simulink model "Tuning"  (R2022b)
settings: Solver=VariableStepAuto  StartTime=0.0  StopTime=100.03  RelTol=1e-3
undefined symbols (not defined in the file): A_matrix, B_matrix, C_matrix, D_matrix, dis_vec, rho_new, sigbuilder_block
libraries: slpidlib x1
settings Model: Creator=brianlesko  LastModifiedBy=brianlesko

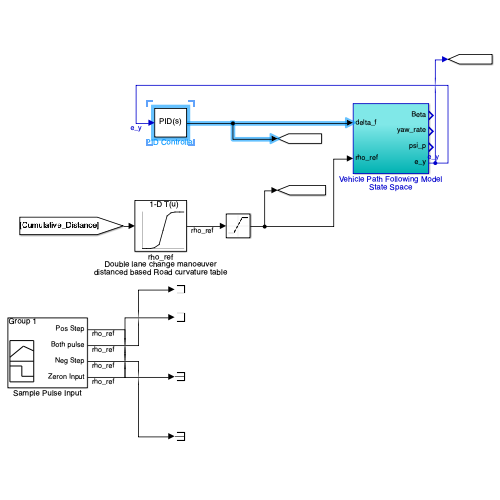
[thumbnail: Simulink's stored preview of the top-level diagram]
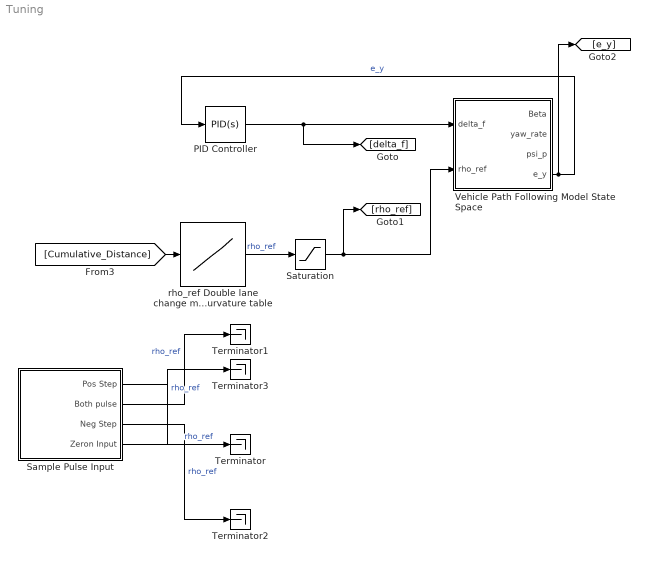
== system Tuning ==
  PID Controller : slpidlib/PID Controller  Controller=PID  Form=Parallel  TimeDomain=Continuous-time  UseExternalTs=off  SampleTime=-1  IntegratorMethod=Forward Euler  FilterMethod=Forward Euler  ControllerParametersSource=internal  P=1.6757e-08  I=1.1959e-08  UseKiTs=off  D=8.9738e-10  N=30  UseFilter=on  TunerSelectOption=Frequency Response Based  InitialConditionSource=internal  InitialConditionForIntegrator=0  InitialConditionForFilter=0  DifferentiatorICPrevScaledInput=0  ExternalReset=none  TrackingMode=off  Kt=1  LimitOutput=off  SatLimitsSource=internal  UpperSaturationLimit=inf  LowerSaturationLimit=-inf  LinearizeAsGain=on  AntiWindupMode=none  Kb=1  LimitIntegrator=off  UpperIntegratorSaturationLimit=inf  LowerIntegratorSaturationLimit=-inf  POutMin=[]  POutMax=[]  IOutMin=[]  IOutMax=[]  DOutMin=[]  DOutMax=[]  NOutMin=[]  NOutMax=[]  SumOutMin=[]  SumOutMax=[]  SaturationOutMin=[]  SaturationOutMax=[]  PParamMin=[]  PParamMax=[]  IParamMin=[]  IParamMax=[]  DParamMin=[]  DParamMax=[]  NParamMin=[]  NParamMax=[]  KbParamMin=[]  KbParamMax=[]  KtParamMin=[]  KtParamMax=[]  KbOutMin=[]  KbOutMax=[]  KtOutMin=[]  KtOutMax=[]  IntegratorOutMin=[]  IntegratorOutMax=[]  FilterOutMin=[]  FilterOutMax=[]  SumI1OutMin=[]  SumI1OutMax=[]  SumI2OutMin=[]  SumI2OutMax=[]  SumI3OutMin=[]  SumI3OutMax=[]  SumI4OutMin=[]  SumI4OutMax=[]  SumDOutMin=[]  SumDOutMax=[]  DifferentiatorOutMin=[]  DifferentiatorOutMax=[]  FilterDiffOutCoefMin=[]  FilterDiffOutCoefMax=[]  ReciprocalOutMin=[]  ReciprocalOutMax=[]  SumDenOutMin=[]  SumDenOutMax=[]  SumNumOutMin=[]  SumNumOutMax=[]  DivideOutMin=[]  DivideOutMax=[]  UdiffTsProdOutMin=[]  UdiffTsProdOutMax=[]  NTsProdOutMin=[]  NTsProdOutMax=[]  UintegralTsProdOutMin=[]  UintegralTsProdOutMax=[]  UngainTsProdOutMin=[]  UngainTsProdOutMax=[]  ClampingZeroOutDataTypeStr=Inherit: Inherit via back propagation  ClampingZeroOutMin=[]  ClampingZeroOutMax=[]  FilterDenConstantOutDataTypeStr=Inherit: Inherit via back propagation  FilterDenConstantOutMin=[]  FilterDenConstantOutMax=[]  PCopyOutDataTypeStr=Inherit: Inherit via back propagation  PCopyOutMin=[]  PCopyOutMax=[]  NCopyOutDataTypeStr=Inherit: Inherit via back propagation  NCopyOutMin=[]  NCopyOutMax=[]  IntegratorContinuousStateAttributes=''  IntegratorStateMustResolveToSignalObject=off  IntegratorRTWStateStorageClass=Auto  FilterContinuousStateAttributes=''  FilterStateMustResolveToSignalObject=off  FilterRTWStateStorageClass=Auto  ParallelPVariant=InternalParameters  IdealPVariant=Disabled  IVariant=InternalParameters  DVariant=InternalParameters  IntegratorVariant=Continuous  SatVariant=Disabled  AWVariant=Passthrough  PCopyVariant=Disabled  TRVariant=Disabled  FdbkBlocksVariant=Forward  IdealPFdbkVariant=Disabled  SatFdbkVariant=Disabled  DerivativeFilterVariant=ContFilter  NVariant=InternalParameters  NCopyVariant=Disabled  FilterICVariant=InternalICsFilter  IntegratorICVariant=InternalICs  ExternalResetVariant=Disabled  TRSumVariant=Passthrough  SumFdbkVariant=Disabled  SumVariant=Sum_PID  TsampFilterVariant=InternalTs  TsampNgainVariant=Passthrough  TsampIntegralVariant=Passthrough  ExternalSaturationOutDataTypeStr=Inherit: Same as second input
  Sample Pulse Input : Subsystem  Tag=STV Subsys  LoadFcn=sigbuilder_block('load');  StartFcn=sigbuilder_block('start');  StopFcn=sigbuilder_block('stop');  ClipboardFcn=sigbuilder_block('clipboard');  mask(Sigbuilder block){tuvar=[0:10]}
      mask help: Simulink:masks:SigbuilderBlock_MD
      mask init:
      | if ~strcmp(get_param(bdroot(gcbh),'SimulationStatus'),'stopped') tuvar = sigbuilder_block('maskInit'); end
      settings: CopyFcn=sigbuilder_block('copy');  DeleteFcn=sigbuilder_block('delete');  ModelCloseFcn=sigbuilder_block('modelClose');  PreSaveFcn=sigbuilder_block('preSave');  PauseFcn=sigbuilder_block('pause');  ContinueFcn=sigbuilder_block('continue');  NameChangeFcn=sigbuilder_block('namechange');  OpenFcn=sigbuilder_block('open',[177 79 1013 454 ]);  CloseFcn=sigbuilder_block('close');
      mask Display: plot(0, 0, 100, 100,[2, 2, 32, 32, 2], [68, 8, 8, 68, 68],[32, 2], [38, 38], [32, 19, 2],[53, 60, 44], [32, 17, 17, 2],[16, 16, 31, 31]);txt = getActiveGroup(gcbh);text(2, 100, txt,'verticalAlignment', 'top');
  Saturation : Saturate  UpperLimit=0.01  LowerLimit=-0.025  LinearizeAsGain=off
  Terminator{,1..3} (4 alike) : Terminator
  Vehicle Path Following Model State Space : Subsystem
  rho_ref Double lane change manoeuver distanced based Road curvature table : Lookup_n-D  NumberOfTableDimensions=1  BreakpointsForDimension1=dis_vec  Table=rho_new  InternalRulePriority=Speed  RndMeth=Simplest
  wires:
  Vehicle Path Following Model State Space/4(e_y) -> PID Controller/1, [e_y]  "e_y"
  Saturation/1 -> Vehicle Path Following Model State Space/2(rho_ref), [rho_ref]
  rho_ref Double lane change manoeuver distanced based Road curvature table/1 -> Saturation/1  "rho_ref"
  [Cumulative_Distance] -> rho_ref Double lane change manoeuver distanced based Road curvature table/1
  Sample Pulse Input/1(Pos Step) -> Terminator/1  "rho_ref"
  Sample Pulse Input/2(Both pulse) -> Terminator1/1  "rho_ref"
  Sample Pulse Input/3(Neg Step) -> Terminator2/1  "rho_ref"
  Sample Pulse Input/4(Zeron Input) -> Terminator3/1  "rho_ref"
  PID Controller/1 -> [delta_f], Vehicle Path Following Model State Space/1(delta_f)

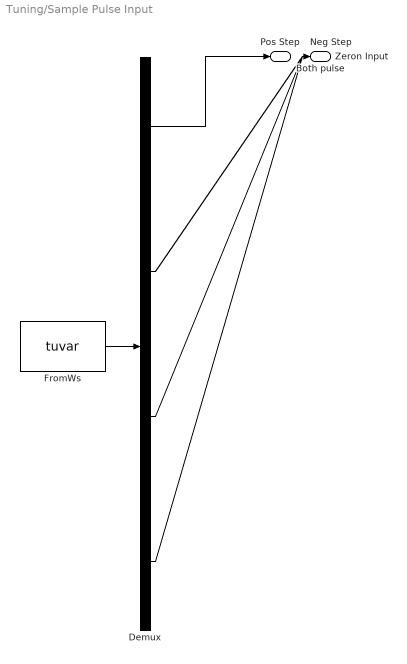
== system Tuning/Sample Pulse Input ==
  Demux : Demux  Tag=STV Demux
      settings: DisplayOption=none
  FromWs : FromWorkspace  Tag=STV FromWs  VariableName=tuvar
      SigBuilderData=|
      | common.afterFinalStr = 'Extrapolate'
      | common.sampleTime = 0
      | dataSet.timeRange = [0 10]
      | dataSet.name = 'Group 1'
      | sbobj.Groups.Name = 'Group 1'
      | sbobj.Groups.Signals(1).Name = 'Pos Step'
      | sbobj.Groups.Signals(1).XData = [0 4 4 6 6 10]
      | sbobj.Groups.Signals(1).YData = [0 0 0.1 0.1 0 0]
      | sbobj.Groups.Signals(2).Name = 'Both pulse'
      | sbobj.Groups.Signals(2).XData = [0 4 4 6 6 7 7 9 9 10]
      | sbobj.Groups.Signals(2).YData = [0 0 0.1 0.1 0 0 -0.1 -0.1 0 0]
      | sbobj.Groups.Signals(3).Name = 'Neg Step'
      | sbobj.Groups.Signals(3).XData = [0 4 4 6 6 10]
      | sbobj.Groups.Signals(3).YData = [0 0 -0.1 -0.1 0 0]
      | sbobj.Groups.Signals(4).Name = 'Zeron Input'
      | sbobj.Groups.Signals(4).XData = [0 10]
      | sbobj.Groups.Signals(4).YData = [0 0]
  Pos Step : Outport  Tag=STV Outport  VectorParamsAs1DForOutWhenUnconnected=off
  Both pulse : Outport  Tag=STV Outport  Port=2  VectorParamsAs1DForOutWhenUnconnected=off
  Neg Step : Outport  Tag=STV Outport  Port=3  VectorParamsAs1DForOutWhenUnconnected=off
  Zeron Input : Outport  Tag=STV Outport  Port=4  VectorParamsAs1DForOutWhenUnconnected=off
  wires:
  FromWs/1 -> Demux/1
  Demux/1 -> Pos Step/1
  Demux/2 -> Both pulse/1
  Demux/3 -> Neg Step/1
  Demux/4 -> Zeron Input/1

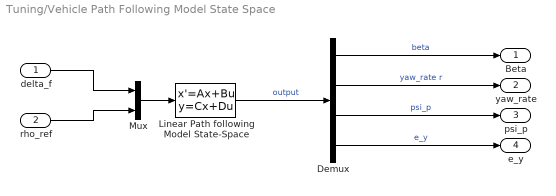
== system Tuning/Vehicle Path Following Model State Space ==
  delta_f : Inport
  rho_ref : Inport  Port=2
  Demux : Demux
  Linear Path following Model State-Space : StateSpace  A=A_matrix  B=B_matrix  C=C_matrix  D=D_matrix  InitialCondition=0
  Mux : Mux  Inputs=2
  Beta : Outport  VectorParamsAs1DForOutWhenUnconnected=off
  yaw_rate : Outport  Port=2  VectorParamsAs1DForOutWhenUnconnected=off
  psi_p : Outport  Port=3  VectorParamsAs1DForOutWhenUnconnected=off
  e_y : Outport  Port=4  VectorParamsAs1DForOutWhenUnconnected=off
  wires:
  Demux/4 -> e_y/1  "e_y"
  Mux/1 -> Linear Path following Model State-Space/1
  Demux/2 -> yaw_rate/1  "yaw_rate r"
  Linear Path following Model State-Space/1 -> Demux/1  "output"
  Demux/1 -> Beta/1  "beta"
  rho_ref/1 -> Mux/2
  delta_f/1 -> Mux/1
  Demux/3 -> psi_p/1  "psi_p"
